simulink model "b"  (R2023a)
settings: Solver=ode4  StartTime=0.0  StopTime=100  FixedStep=0.002  RelTol=1e-3
InitFcn:
  | init;
undefined symbols (not defined in the file or in its folder): attitude_m0, attitude_t0, d_state_m, d_state_t, g, N, state_m0, state_t0
libraries: matrix_library x1, simulink x1
settings Model: Creator=Ali  LastModifiedBy=Ali
settings OptimizationCC: ReuseModelBlockBuffer=off

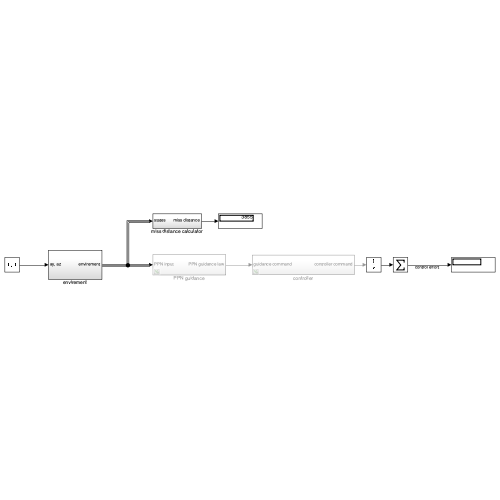
[thumbnail: Simulink's stored preview of the top-level diagram]
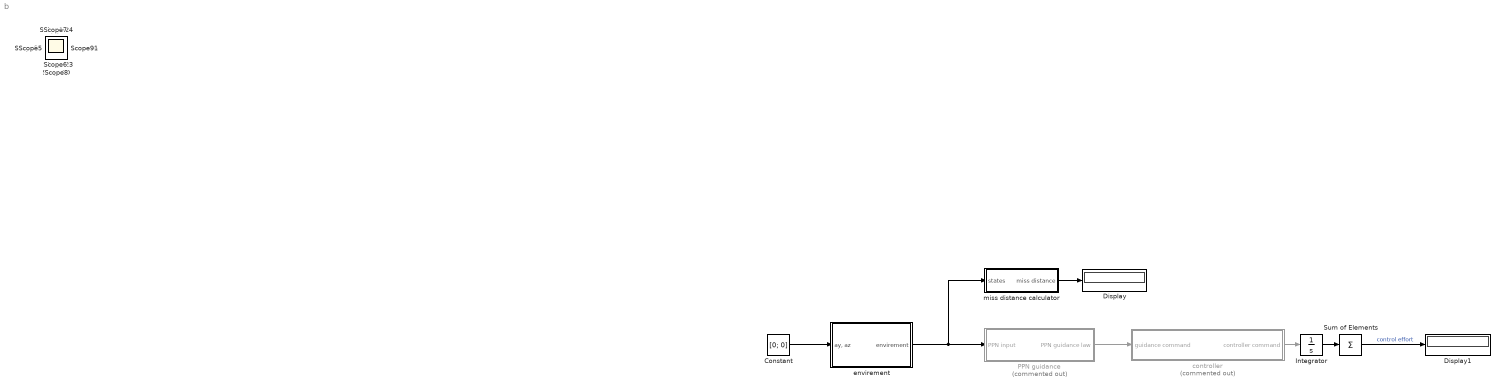
== system b ==
  Constant : Constant  Value=[0; 0]
  Display : Display
  Display1 : Display
  Integrator : Integrator
  PPN guidance : Subsystem  Commented=on
  Sum of Elements : Sum  Inputs=+
  controller : Subsystem  Commented=on
  envirement : Subsystem
  miss distance calculator : Subsystem
  Scope{,1..18,20..24} (24 alike) : Scope
  wires:
  envirement/1(envirement) -> miss distance calculator/1(states), PPN guidance/1(PPN input)
  PPN guidance/1(PPN guidance law) -> controller/1(guidance command)
  miss distance calculator/1(miss distance) -> Display/1
  Constant/1 -> envirement/1("ay, az")
  controller/1(controller command) -> Integrator/1
  Integrator/1 -> Sum of Elements/1
  Sum of Elements/1 -> Display1/1  "control effort"

== system b/PPN guidance ==
  PPN input : Inport
  Bus Selector1 : BusSelector  OutputSignals=missle.missle V,missle.missle attitude,missle.missle satet,missle.misse V_Gl,target.target state,target.target V_G
  Subsystem : Subsystem
  PPN guidance law : Outport
  wires:
  PPN input/1 -> Bus Selector1/1
  Bus Selector1/4 -> Subsystem/4(v_m)  "<misse V_Gl>"
  Bus Selector1/1 -> Subsystem/1(V)  "<missle V>"
  Bus Selector1/5 -> Subsystem/5(state_t)  "<target state>"
  Bus Selector1/6 -> Subsystem/6(v_t)  "<target V_G>"
  Bus Selector1/2 -> Subsystem/2(attitude_m)  "<missle attitude>"
  Bus Selector1/3 -> Subsystem/3(state_m)  "<missle satet>"
  Subsystem/1(PPN) -> PPN guidance law/1

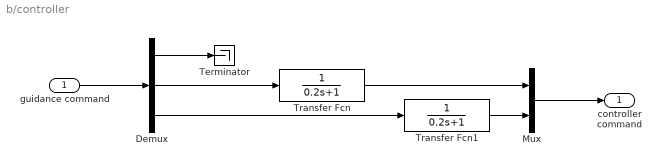
== system b/controller ==
  guidance command : Inport
  Demux : Demux  Outputs=3
  Mux : Mux  Inputs=2
  Terminator : Terminator
  Transfer Fcn : TransferFcn  Denominator=[0.2 1]
  Transfer Fcn1 : TransferFcn  Denominator=[0.2 1]
  controller command : Outport
  wires:
  guidance command/1 -> Demux/1
  Mux/1 -> controller command/1
  Transfer Fcn1/1 -> Mux/2
  Demux/2 -> Transfer Fcn/1
  Demux/1 -> Terminator/1
  Transfer Fcn/1 -> Mux/1
  Demux/3 -> Transfer Fcn1/1

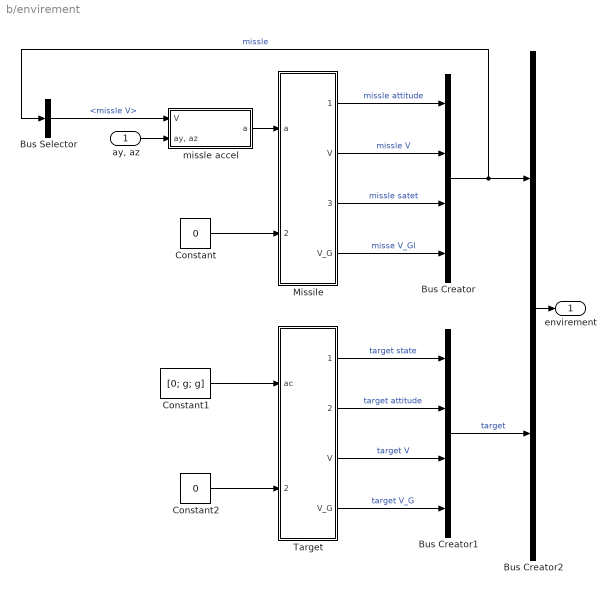
== system b/envirement ==
  "ay, az" : Inport
  Bus Creator : BusCreator  Inputs=4
  Bus Creator1 : BusCreator  Inputs=4
  Bus Creator2 : BusCreator  Inputs=2
  Bus Selector : BusSelector  OutputSignals=missle V
  Constant : Constant  Value=0
  Constant1 : Constant  Value=[0; g; g]
  Constant2 : Constant  Value=0
  "Missile " : Subsystem
  Target : Subsystem
  missle accel : Subsystem
  envirement : Outport
  wires:
  "Missile "/1(attitude) -> Bus Creator/1  "missle attitude"
  Target/2(attitude) -> Bus Creator1/2  "target attitude"
  Target/3(V) -> Bus Creator1/3  "target V"
  "Missile "/2(V) -> Bus Creator/2  "missle V"
  Bus Creator2/1 -> envirement/1
  Target/1(state) -> Bus Creator1/1  "target state"
  "Missile "/4(V_G) -> Bus Creator/4  "misse V_Gl"
  Target/4(V_G) -> Bus Creator1/4  "target V_G"
  Bus Creator1/1 -> Bus Creator2/2  "target"
  Constant2/1 -> Target/2(g_effect)
  Constant1/1 -> Target/1(ac)
  "Missile "/3(state) -> Bus Creator/3  "missle satet"
  missle accel/1(a) -> "Missile "/1(a)
  Constant/1 -> "Missile "/2(g_effect)
  Bus Creator/1 -> Bus Selector/1, Bus Creator2/1  "missle"
  Bus Selector/1 -> missle accel/1(V)  "<missle V>"
  "ay, az"/1 -> missle accel/2("ay, az")

== system b/miss distance calculator ==
  states : Inport
  Bus Selector : BusSelector  OutputSignals=missle.missle satet,target.target state
  miss distance compact : Subsystem
  miss distance : Outport
  wires:
  states/1 -> Bus Selector/1
  miss distance compact/1(miss distance) -> miss distance/1
  Bus Selector/2 -> miss distance compact/2(target)  "<target state>"
  Bus Selector/1 -> miss distance compact/1(missle)  "<missle satet>"

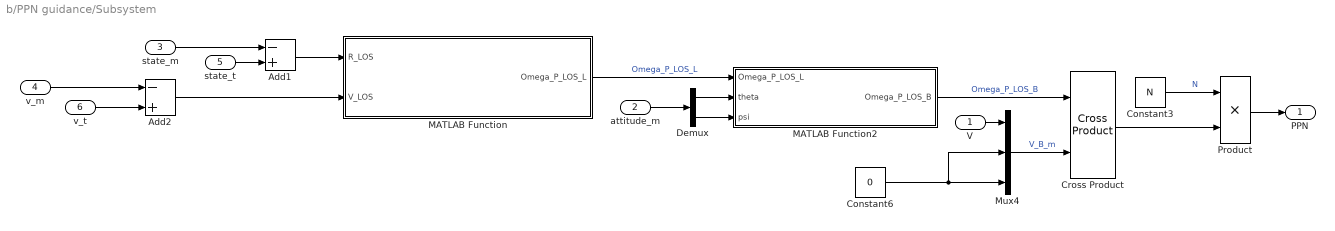
== system b/PPN guidance/Subsystem ==
  V : Inport
  attitude_m : Inport  Port=2
  state_m : Inport  Port=3
  v_m : Inport  Port=4
  state_t : Inport  Port=5
  v_t : Inport  Port=6
  Add1 : Sum  Inputs=-+
  Add2 : Sum  Inputs=-+
  Constant3 : Constant  Value=N
  Constant6 : Constant  Value=0
  Cross Product : matrix_library/Cross Product
  Demux : Demux  Outputs=2
  MATLAB Function : MATLAB Function  TreatAsAtomicUnit=on
  MATLAB Function2 : MATLAB Function  TreatAsAtomicUnit=on
  Mux4 : Mux  Inputs=3
  Product : Product
  PPN : Outport
  wires:
  state_t/1 -> Add1/2
  Product/1 -> PPN/1
  V/1 -> Mux4/1
  Demux/2 -> MATLAB Function2/3(psi)
  v_m/1 -> Add2/1
  Add1/1 -> MATLAB Function/1(R_LOS)
  Constant3/1 -> Product/1  "N"
  Add2/1 -> MATLAB Function/2(V_LOS)
  attitude_m/1 -> Demux/1
  v_t/1 -> Add2/2
  MATLAB Function/1(Omega_P_LOS_L) -> MATLAB Function2/1(Omega_P_LOS_L)  "Omega_P_LOS_L"
  Constant6/1 -> Mux4/2, Mux4/3
  Mux4/1 -> Cross Product/2  "V_B_m"
  state_m/1 -> Add1/1
  Demux/1 -> MATLAB Function2/2(theta)
  Cross Product/1 -> Product/2
  MATLAB Function2/1(Omega_P_LOS_B) -> Cross Product/1  "Omega_P_LOS_B"

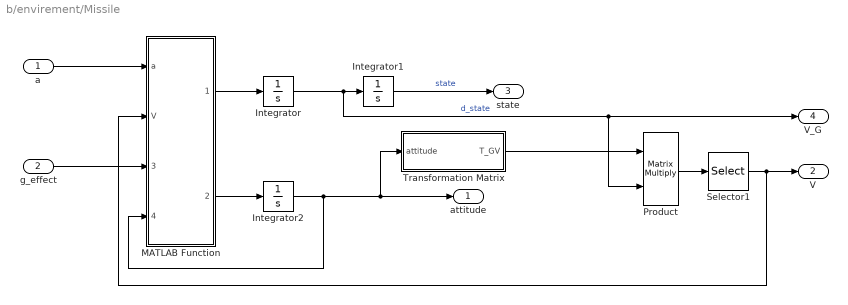
== system b/envirement/Missile  ==
  a : Inport
  g_effect : Inport  Port=2
  Integrator : Integrator  InitialCondition=d_state_m
  Integrator1 : Integrator  InitialCondition=state_m0
  Integrator2 : Integrator  InitialCondition=attitude_m0
  MATLAB Function : MATLAB Function  TreatAsAtomicUnit=on
  Product : Product  Multiplication=Matrix(*)
  Selector1 : Selector  InputPortWidth=3  IndexOptions=Index vector (dialog)  Indices=[1]  OutputSizes=1
  Transformation Matrix : MATLAB Function  TreatAsAtomicUnit=on
  attitude : Outport
  V : Outport  Port=2
  state : Outport  Port=3
  V_G : Outport  Port=4
  wires:
  MATLAB Function/2(dot_attitude) -> Integrator2/1
  Integrator1/1 -> state/1  "state"
  MATLAB Function/1(dd_state) -> Integrator/1
  g_effect/1 -> MATLAB Function/3(g_effect)
  Integrator/1 -> Integrator1/1, Product/2, V_G/1  "d_state"
  Product/1 -> Selector1/1
  Selector1/1 -> MATLAB Function/2(V), V/1
  Integrator2/1 -> Transformation Matrix/1(attitude), attitude/1, MATLAB Function/4(attitude)
  a/1 -> MATLAB Function/1(a)
  Transformation Matrix/1(T_GV) -> Product/1

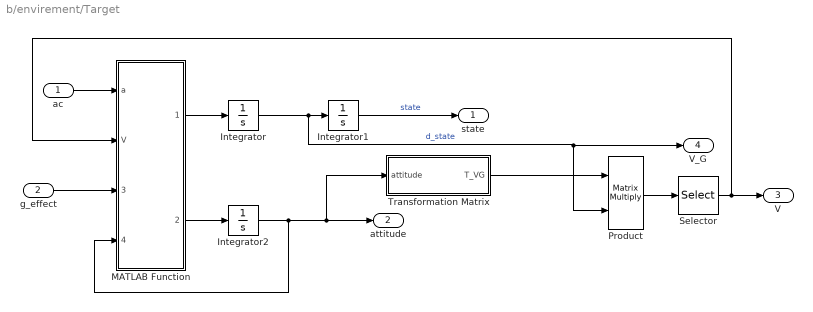
== system b/envirement/Target ==
  ac : Inport
  g_effect : Inport  Port=2
  Integrator : Integrator  InitialCondition=d_state_t
  Integrator1 : Integrator  InitialCondition=state_t0
  Integrator2 : Integrator  InitialCondition=attitude_t0
  MATLAB Function : MATLAB Function  TreatAsAtomicUnit=on
  Product : Product  Multiplication=Matrix(*)
  Selector : Selector  InputPortWidth=3  IndexOptions=Index vector (dialog)  Indices=[1]  OutputSizes=1
  Transformation Matrix : MATLAB Function  TreatAsAtomicUnit=on
  state : Outport
  attitude : Outport  Port=2
  V : Outport  Port=3
  V_G : Outport  Port=4
  wires:
  MATLAB Function/2(dot_attitude) -> Integrator2/1
  Integrator1/1 -> state/1  "state"
  MATLAB Function/1(dd_state) -> Integrator/1
  g_effect/1 -> MATLAB Function/3(g_effect)
  Integrator/1 -> V_G/1, Product/2, Integrator1/1  "d_state"
  Integrator2/1 -> MATLAB Function/4(attitude), Transformation Matrix/1(attitude), attitude/1
  Product/1 -> Selector/1
  Selector/1 -> MATLAB Function/2(V), V/1
  ac/1 -> MATLAB Function/1(a)
  Transformation Matrix/1(T_VG) -> Product/1

== system b/envirement/missle accel ==
  V : Inport
  "ay, az" : Inport  Port=2
  Mux : Mux  Inputs=2
  acceleration : Subsystem
  a : Outport
  wires:
  Mux/1 -> a/1
  V/1 -> acceleration/1(V)
  acceleration/1(ax) -> Mux/1
  "ay, az"/1 -> Mux/2

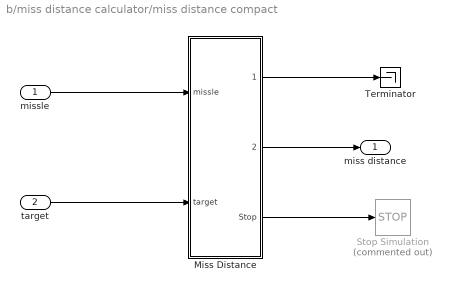
== system b/miss distance calculator/miss distance compact ==
  missle : Inport
  target : Inport  Port=2
  Miss Distance : Subsystem
  Stop Simulation : Stop  Commented=on
  Terminator : Terminator
  miss distance : Outport
  wires:
  target/1 -> Miss Distance/2(target)
  Miss Distance/1(distance) -> Terminator/1
  Miss Distance/2(miss distance) -> miss distance/1
  missle/1 -> Miss Distance/1(missle)
  Miss Distance/3(Stop) -> Stop Simulation/1

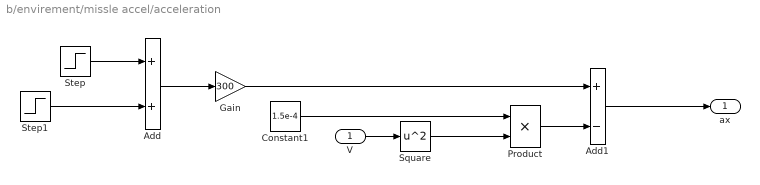
== system b/envirement/missle accel/acceleration ==
  V : Inport
  Add : Sum
  Add1 : Sum  Inputs=+-
  Constant1 : Constant  Value=1.5e-4
  Gain : Gain  Gain=300
  Product : Product
  Square : Math  Operator=square
  Step : Step  Time=3  After=-1  SampleTime=0
  Step1 : Step  Time=0  SampleTime=0
  ax : Outport
  wires:
  V/1 -> Square/1
  Step/1 -> Add/1
  Square/1 -> Product/2
  Constant1/1 -> Product/1
  Add1/1 -> ax/1
  Step1/1 -> Add/2
  Gain/1 -> Add1/1
  Add/1 -> Gain/1
  Product/1 -> Add1/2

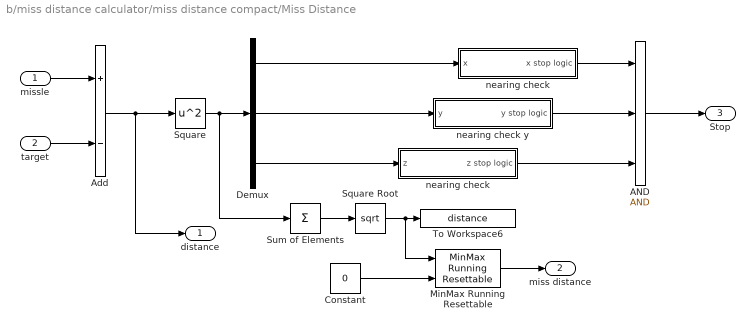
== system b/miss distance calculator/miss distance compact/Miss Distance ==
  missle : Inport
  target : Inport  Port=2
  AND : Logic  Inputs=3  IconShape=distinctive  AllPortsSameDT=off  OutDataTypeStr=boolean
  Add : Sum  Inputs=+-
  Constant : Constant  Value=0
  Demux : Demux  Outputs=3
  MinMax Running Resettable : simulink/Math Operations/MinMax Running Resettable  Function=min  vinit=inf
  Square : Math  Operator=square
  Square Root : Sqrt
  Sum of Elements : Sum  Inputs=+
  To Workspace6 : ToWorkspace  VariableName=distance  SaveFormat=Timeseries  SampleTime=-1
      settings: Save2DSignal=2-D array (concatenate along first dimension)
  nearing check : Subsystem
  "nearing check " : Subsystem
  nearing check y : Subsystem
  distance : Outport
  miss distance : Outport  Port=2
  Stop : Outport  Port=3
  wires:
  missle/1 -> Add/1
  Add/1 -> distance/1, Square/1
  target/1 -> Add/2
  Square/1 -> Sum of Elements/1, Demux/1
  nearing check/1(x stop logic) -> AND/1
  AND/1 -> Stop/1
  Demux/2 -> nearing check y/1(y)
  Sum of Elements/1 -> Square Root/1
  Square Root/1 -> MinMax Running Resettable/1, To Workspace6/1
  Demux/3 -> "nearing check "/1(z)
  Demux/1 -> nearing check/1(x)
  Constant/1 -> MinMax Running Resettable/2
  MinMax Running Resettable/1 -> miss distance/1
  "nearing check "/1(z stop logic) -> AND/3
  nearing check y/1(y stop logic) -> AND/2

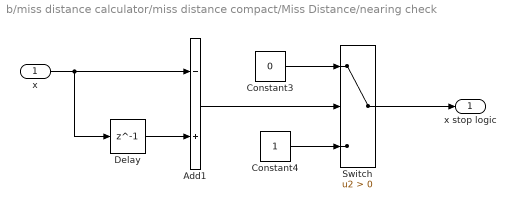
== system b/miss distance calculator/miss distance compact/Miss Distance/nearing check ==
  x : Inport
  Add1 : Sum  Inputs=-+
  Constant3 : Constant  Value=0
  Constant4 : Constant
  Delay : Delay  DelayLength=1  InitialCondition=inf
  Switch : Switch  Criteria=u2 > Threshold  SaturateOnIntegerOverflow=off  InputSameDT=off
  x stop logic : Outport
  wires:
  Switch/1 -> x stop logic/1
  Constant3/1 -> Switch/1
  Constant4/1 -> Switch/3
  x/1 -> Delay/1, Add1/1
  Add1/1 -> Switch/2
  Delay/1 -> Add1/2

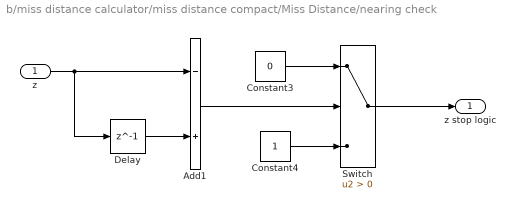
== system b/miss distance calculator/miss distance compact/Miss Distance/nearing check  ==
  z : Inport
  Add1 : Sum  Inputs=-+
  Constant3 : Constant  Value=0
  Constant4 : Constant
  Delay : Delay  DelayLength=1  InitialCondition=inf
  Switch : Switch  Criteria=u2 > Threshold  SaturateOnIntegerOverflow=off  InputSameDT=off
  z stop logic : Outport
  wires:
  Delay/1 -> Add1/2
  Add1/1 -> Switch/2
  z/1 -> Add1/1, Delay/1
  Constant4/1 -> Switch/3
  Constant3/1 -> Switch/1
  Switch/1 -> z stop logic/1

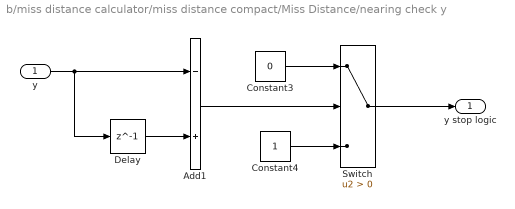
== system b/miss distance calculator/miss distance compact/Miss Distance/nearing check y ==
  y : Inport
  Add1 : Sum  Inputs=-+
  Constant3 : Constant  Value=0
  Constant4 : Constant
  Delay : Delay  DelayLength=1  InitialCondition=inf
  Switch : Switch  Criteria=u2 > Threshold  SaturateOnIntegerOverflow=off  InputSameDT=off
  y stop logic : Outport
  wires:
  Delay/1 -> Add1/2
  Add1/1 -> Switch/2
  y/1 -> Add1/1, Delay/1
  Constant4/1 -> Switch/3
  Constant3/1 -> Switch/1
  Switch/1 -> y stop logic/1

== matlab function b/envirement/Missile /Transformation Matrix ==
  data: attitude input; T_GV output
function T_GV = fcn(attitude)
theta = attitude(1);
psi = attitude(2);

T_GV = [cos(theta)*cos(psi)   cos(theta)*sin(psi)   sin(theta)
            -sin(psi)               cos(psi)            0
        -sin(theta)*cos(psi)  -sin(theta)*sin(psi)   cos(theta) ];

== matlab function b/envirement/Missile /MATLAB Function ==
  data: a input; dd_state output; V input; g_effect input; attitude input; dot_attitude output
function [dd_state, dot_attitude] =...
    fcn(a, V, g_effect, attitude)
a_x = a(1);
a_y = a(2);
a_z = a(3);

theta = attitude(1);
psi = attitude(2);
g = 9.81;
g = g*g_effect;

ddot_x = a_x*cos(theta)*cos(psi) - a_y*sin(psi) - a_z*sin(theta)*cos(psi);
ddot_y = a_x*cos(theta)*sin(psi) + a_y*cos(psi) - a_z*sin(theta)*sin(psi);
ddot_z = a_x*sin(theta) + a_z*cos(theta) - g;

dd_state = [ddot_x; ddot_y; ddot_z];

dot_theta = (a_z - g*cos(theta)) / V;
dot_psi   = a_y / (V*cos(theta));

dot_attitude = [dot_theta; dot_psi];

== matlab function b/envirement/Target/MATLAB Function ==
  data: a input; dd_state output; V input; g_effect input; attitude input; dot_attitude output
function [dd_state, dot_attitude] =...
    fcn(a, V, g_effect, attitude)
a_x = a(1);
a_y = a(2);
a_z = a(3);

theta = attitude(1);
psi = attitude(2);
g = 9.81;
g = g*g_effect;

ddot_x = a_x*cos(theta)*cos(psi) - a_y*sin(psi) - a_z*sin(theta)*cos(psi);
ddot_y = a_x*cos(theta)*sin(psi) + a_y*cos(psi) - a_z*sin(theta)*sin(psi);
ddot_z = a_x*sin(theta) + a_z*cos(theta) - g;

dd_state = [ddot_x; ddot_y; ddot_z];

g = 9.81;
dot_theta = (a_z - g*cos(theta)) / V;
dot_psi   = a_y / (V*cos(theta));

dot_attitude = [dot_theta; dot_psi];

== matlab function b/envirement/Target/Transformation Matrix ==
  data: attitude input; T_VG output
function T_VG = fcn(attitude)
theta = attitude(1);
psi = attitude(2);

T_VG = [cos(theta)*cos(psi)   cos(theta)*sin(psi)   sin(theta)
            -sin(psi)               cos(psi)            0
        -sin(theta)*cos(psi)  -sin(theta)*sin(psi)   cos(theta) ];

== matlab function b/PPN guidance/Subsystem/MATLAB Function ==
  data: R_LOS input; Omega_P_LOS_L output; V_LOS input
function Omega_P_LOS_L = omega_calculator(R_LOS,V_LOS)
%definning skew symetric matrix of R for cross product
R_skew_sym = [   0        -R_LOS(3)     R_LOS(2)
               R_LOS(3)      0         -R_LOS(1)
              -R_LOS(2)    R_LOS(1)        0     ];

%norm of R
norm_R = R_LOS(1)^2 + R_LOS(2)^2 +R_LOS(3)^2;

%Omega Perpendicular LOS in Local Level cordinate system
Omega_P_LOS_L = R_skew_sym*V_LOS/norm_R;

== matlab function b/PPN guidance/Subsystem/MATLAB Function2 ==
  data: Omega_P_LOS_L input; theta input; Omega_P_LOS_B output; psi input
function Omega_P_LOS_B = T_B_L(Omega_P_LOS_L,theta,psi)

T_B_L = [cos(theta)*cos(psi)   cos(theta)*sin(psi)   sin(theta)
            -sin(psi)               cos(psi)            0
        -sin(theta)*cos(psi)  -sin(theta)*sin(psi)   cos(theta) ];

Omega_P_LOS_B = T_B_L*Omega_P_LOS_L;
end
